simulink model "physicalmodel"  (R2025b)
settings: Solver=VariableStepAuto  StartTime=0.0  StopTime=10.0  RelTol=1e-3
model workspace: external: MATLAB File G:\My Drive\SimSys\Zadania\Zadanie c.4\Create_hydraulic1_model.m (data not in the file)
settings Model: Creator=arxchy  LastModifiedBy=arxchy

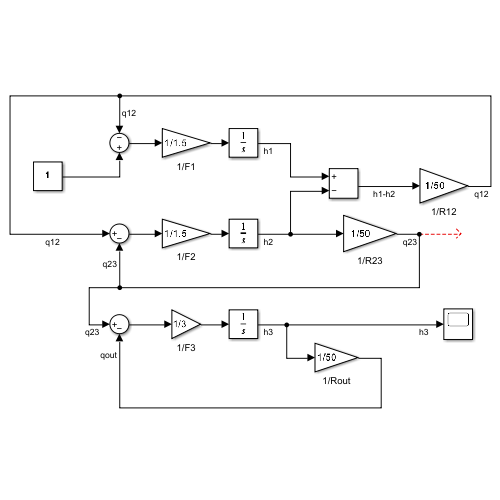
[thumbnail: Simulink's stored preview of the top-level diagram]
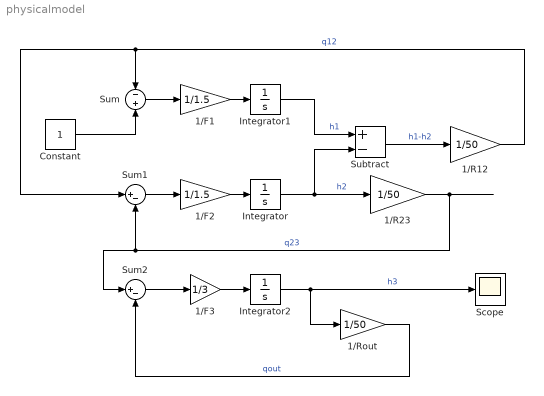
== system physicalmodel ==
  1/F1 : Gain  Gain=1/1.5
  1/F2 : Gain  Gain=1/1.5
  1/F3 : Gain  Gain=1/3
  1/R12 : Gain  Gain=1/50
  1/R23 : Gain  Gain=1/50
  1/Rout : Gain  Gain=1/50
  Constant : Constant
  Integrator : Integrator
  Integrator1 : Integrator
  Integrator2 : Integrator
  Scope : Scope
      settings: ActiveDisplayYMinimum=-0.0011006337977021929  ActiveDisplayYMaximum=0.0099057041793197374
  Subtract : Sum  Inputs=+-
  Sum : Sum  Inputs=-+
  Sum1 : Sum  Inputs=|+-
  Sum2 : Sum  Inputs=|+-
  wires:
  Integrator1/1 -> Subtract/1  "h1"
  Integrator/1 -> Subtract/2, 1/R23/1  "h2"
  Integrator2/1 -> 1/Rout/1, Scope/1  "h3"
  Subtract/1 -> 1/R12/1  "h1-h2"
  1/R12/1 -> Sum1/1, Sum/1  "q12"
  1/R23/1 -> Sum2/1, Sum1/2  "q23"
  1/Rout/1 -> Sum2/2  "qout"
  Sum/1 -> 1/F1/1
  1/F1/1 -> Integrator1/1
  Constant/1 -> Sum/2
  1/F2/1 -> Integrator/1
  Sum1/1 -> 1/F2/1
  1/F3/1 -> Integrator2/1
  Sum2/1 -> 1/F3/1
